simulink model "Matematicki_model_final"  (R2018a)
settings: Solver=ode45  StartTime=0.0  StopTime=60  FixedStep=0.01  RelTol=1e-3
libraries: slident x1
settings Model: Creator=Zeljko  LastModifiedBy=Zeljko

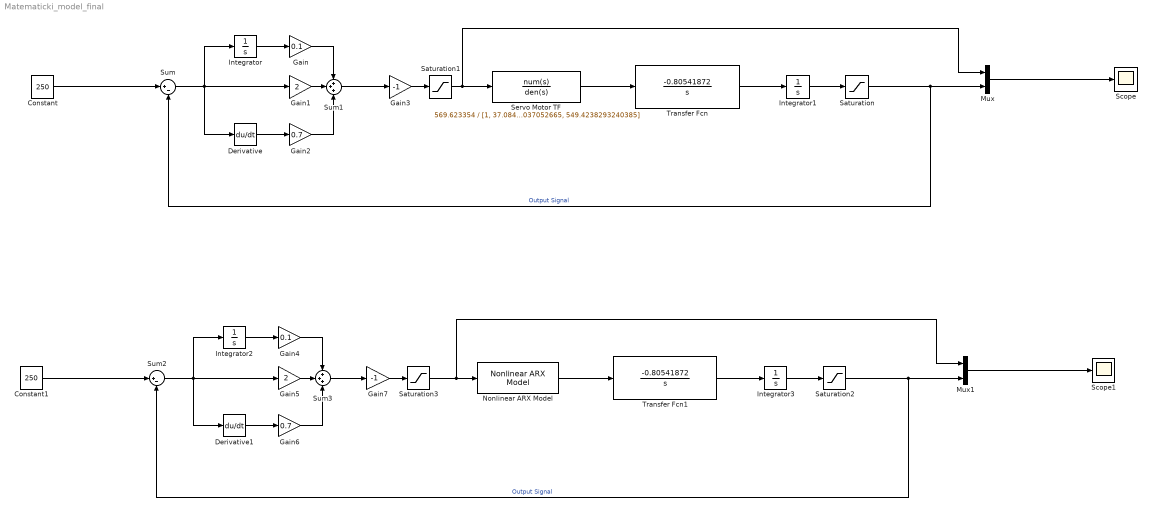
== system Matematicki_model_final ==
  Constant : Constant  Value=250
  Constant1 : Constant  Value=250
  Derivative : Derivative
  Derivative1 : Derivative
  Gain : Gain  Gain=0.1
  Gain1 : Gain  Gain=2
  Gain2 : Gain  Gain=0.7
  Gain3 : Gain  Gain=-1
  Gain4 : Gain  Gain=0.1
  Gain5 : Gain  Gain=2
  Gain6 : Gain  Gain=0.7
  Gain7 : Gain  Gain=-1
  Integrator : Integrator
  Integrator1 : Integrator  InitialCondition=330
  Integrator2 : Integrator
  Integrator3 : Integrator  InitialCondition=330
  Mux : Mux  Inputs=2
  Mux1 : Mux  Inputs=2
  Nonlinear ARX Model : slident/Models/Nonlinear ARX Model  sys=sys  ICspec=State values  X0=[0;0;0;0;0;0;0]  U0=0  Y0=0
      settings: SourceProductName=System Identification Toolbox  SourceProductBaseCode=ID
  Saturation : Saturate  UpperLimit=400  LowerLimit=0
  Saturation1 : Saturate  UpperLimit=30  LowerLimit=-30
  Saturation2 : Saturate  UpperLimit=400  LowerLimit=0
  Saturation3 : Saturate  UpperLimit=30  LowerLimit=-30
  Scope : Scope
  Scope1 : Scope
  Servo Motor TF : TransferFcn  Numerator=569.623354  Denominator=[1, 37.084598037052665, 549.4238293240385]
  Sum : Sum  Inputs=|+-
  Sum1 : Sum  Inputs=+++
  Sum2 : Sum  Inputs=|+-
  Sum3 : Sum  Inputs=+++
  Transfer Fcn : TransferFcn  Numerator=-0.80541872  Denominator=[1 0]
  Transfer Fcn1 : TransferFcn  Numerator=-0.80541872  Denominator=[1 0]
  wires:
  Sum/1 -> Derivative/1, Integrator/1, Gain1/1
  Integrator/1 -> Gain/1
  Gain/1 -> Sum1/1
  Gain2/1 -> Sum1/3
  Gain1/1 -> Sum1/2
  Derivative/1 -> Gain2/1
  Saturation/1 -> Mux/2, Sum/2  "Output Signal"
  Saturation1/1 -> Mux/1, Servo Motor TF/1
  Constant/1 -> Sum/1
  Mux/1 -> Scope/1
  Transfer Fcn/1 -> Integrator1/1
  Integrator1/1 -> Saturation/1
  Sum1/1 -> Gain3/1
  Gain3/1 -> Saturation1/1
  Servo Motor TF/1 -> Transfer Fcn/1
  Saturation2/1 -> Mux1/2, Sum2/2  "Output Signal"
  Saturation3/1 -> Nonlinear ARX Model/1, Mux1/1
  Sum3/1 -> Gain7/1
  Constant1/1 -> Sum2/1
  Mux1/1 -> Scope1/1
  Derivative1/1 -> Gain6/1
  Nonlinear ARX Model/1 -> Transfer Fcn1/1
  Gain5/1 -> Sum3/2
  Integrator2/1 -> Gain4/1
  Transfer Fcn1/1 -> Integrator3/1
  Sum2/1 -> Derivative1/1, Integrator2/1, Gain5/1
  Gain7/1 -> Saturation3/1
  Gain6/1 -> Sum3/3
  Integrator3/1 -> Saturation2/1
  Gain4/1 -> Sum3/1
